simulink model "P702_NI_SoftECU"  (R2019a)
settings: Solver=ode1  StartTime=0.0  StopTime=Inf  FixedStep=0.001  RelTol=1e-3  EnableMultiTasking=on
PreLoadFcn:
  | run '.\VeriStand_BlockSet\NIVeriStandAddPaths.m'
undefined symbols (not defined in the file or in its folder): magnitude
libraries: simulink x83, simulink_extras x1
(part 47 of 76)

== system P702_NI_SoftECU/Input/GWM-SCCM//PDB//RCM//GSM/Other_GWMTx/Driver_Dr_Stat_FD1 ==
  BLISLEDStatDriverSide : S-Function  Priority=1  FunctionName=NIVeriStandIO  Parameters=width dtype portnum stime stype btype  SFunctionDeploymentMode=off  EnableBusSupport=off  mask(NI VeriStand Inport){portnum=1, width=-1, stime=-1, dtype=auto, stype=auto, btype=1}
      mask prompts: portnum "Port number:"; width "Port dimensions (-1 for dynamically sized):"; stime "Sample time (-1 for inherited):"; dtype "Data type:"; stype "Signal type:"; btype "Block type:"
      mask help: Use this inport on any level of nested subsystems to allow NI VeriStand software to map signals to it.
      mask init:
      | NIVeriStandIO_init;
      settings: CopyFcn=NIVeriStand_MDL_functions('', 'IO_copy');  DeleteFcn=NIVeriStand_MDL_functions('', 'IO_delete');  MoveFcn=set_param(gcb, 'Mask', 'on');
      mask Callback portnum: NIVeriStand_MDL_functions('', 'IO_setportnum');
      mask TypeOptions dtype: auto | double | single | int8 | uint8 | int16 | uint16 | int32 | uint32 | boolean
      mask Callback dtype: NIVeriStand_MDL_functions('', 'IO_booleansignal');
      mask TypeOptions stype: auto | real | complex
      mask Display:
      | patch([-x x], [-y y], [.90980 .81960 .32156]);
      | plot([xrad -x x xrad], [yrad -y y yrad]);
      | fprintf('NI In%d', portnum);
  Bus_Sig : BusCreator  Inputs=10
  ChildLckFdbckRd_B_Stat : S-Function  Priority=2  FunctionName=NIVeriStandIO  Parameters=width dtype portnum stime stype btype  SFunctionDeploymentMode=off  EnableBusSupport=off  mask(NI VeriStand Inport){portnum=2, width=-1, stime=-1, dtype=auto, stype=auto, btype=1}
      mask prompts: portnum "Port number:"; width "Port dimensions (-1 for dynamically sized):"; stime "Sample time (-1 for inherited):"; dtype "Data type:"; stype "Signal type:"; btype "Block type:"
      mask help: Use this inport on any level of nested subsystems to allow NI VeriStand software to map signals to it.
      mask init:
      | NIVeriStandIO_init;
      settings: CopyFcn=NIVeriStand_MDL_functions('', 'IO_copy');  DeleteFcn=NIVeriStand_MDL_functions('', 'IO_delete');  MoveFcn=set_param(gcb, 'Mask', 'on');
      mask Callback portnum: NIVeriStand_MDL_functions('', 'IO_setportnum');
      mask TypeOptions dtype: auto | double | single | int8 | uint8 | int16 | uint16 | int32 | uint32 | boolean
      mask Callback dtype: NIVeriStand_MDL_functions('', 'IO_booleansignal');
      mask TypeOptions stype: auto | real | complex
      mask Display:
      | patch([-x x], [-y y], [.90980 .81960 .32156]);
      | plot([xrad -x x xrad], [yrad -y y yrad]);
      | fprintf('NI In%d', portnum);
  ChildLckPw_D_Rq : S-Function  Priority=3  FunctionName=NIVeriStandIO  Parameters=width dtype portnum stime stype btype  SFunctionDeploymentMode=off  EnableBusSupport=off  mask(NI VeriStand Inport){portnum=3, width=-1, stime=-1, dtype=auto, stype=auto, btype=1}
      mask prompts: portnum "Port number:"; width "Port dimensions (-1 for dynamically sized):"; stime "Sample time (-1 for inherited):"; dtype "Data type:"; stype "Signal type:"; btype "Block type:"
      mask help: Use this inport on any level of nested subsystems to allow NI VeriStand software to map signals to it.
      mask init:
      | NIVeriStandIO_init;
      settings: CopyFcn=NIVeriStand_MDL_functions('', 'IO_copy');  DeleteFcn=NIVeriStand_MDL_functions('', 'IO_delete');  MoveFcn=set_param(gcb, 'Mask', 'on');
      mask Callback portnum: NIVeriStand_MDL_functions('', 'IO_setportnum');
      mask TypeOptions dtype: auto | double | single | int8 | uint8 | int16 | uint16 | int32 | uint32 | boolean
      mask Callback dtype: NIVeriStand_MDL_functions('', 'IO_booleansignal');
      mask TypeOptions stype: auto | real | complex
      mask Display:
      | patch([-x x], [-y y], [.90980 .81960 .32156]);
      | plot([xrad -x x xrad], [yrad -y y yrad]);
      | fprintf('NI In%d', portnum);
  ChildLckPw_N_Cnt : S-Function  Priority=4  FunctionName=NIVeriStandIO  Parameters=width dtype portnum stime stype btype  SFunctionDeploymentMode=off  EnableBusSupport=off  mask(NI VeriStand Inport){portnum=4, width=-1, stime=-1, dtype=auto, stype=auto, btype=1}
      mask prompts: portnum "Port number:"; width "Port dimensions (-1 for dynamically sized):"; stime "Sample time (-1 for inherited):"; dtype "Data type:"; stype "Signal type:"; btype "Block type:"
      mask help: Use this inport on any level of nested subsystems to allow NI VeriStand software to map signals to it.
      mask init:
      | NIVeriStandIO_init;
      settings: CopyFcn=NIVeriStand_MDL_functions('', 'IO_copy');  DeleteFcn=NIVeriStand_MDL_functions('', 'IO_delete');  MoveFcn=set_param(gcb, 'Mask', 'on');
      mask Callback portnum: NIVeriStand_MDL_functions('', 'IO_setportnum');
      mask TypeOptions dtype: auto | double | single | int8 | uint8 | int16 | uint16 | int32 | uint32 | boolean
      mask Callback dtype: NIVeriStand_MDL_functions('', 'IO_booleansignal');
      mask TypeOptions stype: auto | real | complex
      mask Display:
      | patch([-x x], [-y y], [.90980 .81960 .32156]);
      | plot([xrad -x x xrad], [yrad -y y yrad]);
      | fprintf('NI In%d', portnum);
  Driver_Lock_Sw_Cnt : S-Function  Priority=5  FunctionName=NIVeriStandIO  Parameters=width dtype portnum stime stype btype  SFunctionDeploymentMode=off  EnableBusSupport=off  mask(NI VeriStand Inport){portnum=5, width=-1, stime=-1, dtype=auto, stype=auto, btype=1}
      mask prompts: portnum "Port number:"; width "Port dimensions (-1 for dynamically sized):"; stime "Sample time (-1 for inherited):"; dtype "Data type:"; stype "Signal type:"; btype "Block type:"
      mask help: Use this inport on any level of nested subsystems to allow NI VeriStand software to map signals to it.
      mask init:
      | NIVeriStandIO_init;
      settings: CopyFcn=NIVeriStand_MDL_functions('', 'IO_copy');  DeleteFcn=NIVeriStand_MDL_functions('', 'IO_delete');  MoveFcn=set_param(gcb, 'Mask', 'on');
      mask Callback portnum: NIVeriStand_MDL_functions('', 'IO_setportnum');
      mask TypeOptions dtype: auto | double | single | int8 | uint8 | int16 | uint16 | int32 | uint32 | boolean
      mask Callback dtype: NIVeriStand_MDL_functions('', 'IO_booleansignal');
      mask TypeOptions stype: auto | real | complex
      mask Display:
      | patch([-x x], [-y y], [.90980 .81960 .32156]);
      | plot([xrad -x x xrad], [yrad -y y yrad]);
      | fprintf('NI In%d', portnum);
  Driver_Lock_Sw_Stat : S-Function  Priority=6  FunctionName=NIVeriStandIO  Parameters=width dtype portnum stime stype btype  SFunctionDeploymentMode=off  EnableBusSupport=off  mask(NI VeriStand Inport){portnum=6, width=-1, stime=-1, dtype=auto, stype=auto, btype=1}
      mask prompts: portnum "Port number:"; width "Port dimensions (-1 for dynamically sized):"; stime "Sample time (-1 for inherited):"; dtype "Data type:"; stype "Signal type:"; btype "Block type:"
      mask help: Use this inport on any level of nested subsystems to allow NI VeriStand software to map signals to it.
      mask init:
      | NIVeriStandIO_init;
      settings: CopyFcn=NIVeriStand_MDL_functions('', 'IO_copy');  DeleteFcn=NIVeriStand_MDL_functions('', 'IO_delete');  MoveFcn=set_param(gcb, 'Mask', 'on');
      mask Callback portnum: NIVeriStand_MDL_functions('', 'IO_setportnum');
      mask TypeOptions dtype: auto | double | single | int8 | uint8 | int16 | uint16 | int32 | uint32 | boolean
      mask Callback dtype: NIVeriStand_MDL_functions('', 'IO_booleansignal');
      mask TypeOptions stype: auto | real | complex
      mask Display:
      | patch([-x x], [-y y], [.90980 .81960 .32156]);
      | plot([xrad -x x xrad], [yrad -y y yrad]);
      | fprintf('NI In%d', portnum);
  KeyCylSwDrvDr_D_Stat : S-Function  Priority=7  FunctionName=NIVeriStandIO  Parameters=width dtype portnum stime stype btype  SFunctionDeploymentMode=off  EnableBusSupport=off  mask(NI VeriStand Inport){portnum=7, width=-1, stime=-1, dtype=auto, stype=auto, btype=1}
      mask prompts: portnum "Port number:"; width "Port dimensions (-1 for dynamically sized):"; stime "Sample time (-1 for inherited):"; dtype "Data type:"; stype "Signal type:"; btype "Block type:"
      mask help: Use this inport on any level of nested subsystems to allow NI VeriStand software to map signals to it.
      mask init:
      | NIVeriStandIO_init;
      settings: CopyFcn=NIVeriStand_MDL_functions('', 'IO_copy');  DeleteFcn=NIVeriStand_MDL_functions('', 'IO_delete');  MoveFcn=set_param(gcb, 'Mask', 'on');
      mask Callback portnum: NIVeriStand_MDL_functions('', 'IO_setportnum');
      mask TypeOptions dtype: auto | double | single | int8 | uint8 | int16 | uint16 | int32 | uint32 | boolean
      mask Callback dtype: NIVeriStand_MDL_functions('', 'IO_booleansignal');
      mask TypeOptions stype: auto | real | complex
      mask Display:
      | patch([-x x], [-y y], [.90980 .81960 .32156]);
      | plot([xrad -x x xrad], [yrad -y y yrad]);
      | fprintf('NI In%d', portnum);
  RollCodeDrvDrKeyCyl : S-Function  Priority=8  FunctionName=NIVeriStandIO  Parameters=width dtype portnum stime stype btype  SFunctionDeploymentMode=off  EnableBusSupport=off  mask(NI VeriStand Inport){portnum=8, width=-1, stime=-1, dtype=auto, stype=auto, btype=1}
      mask prompts: portnum "Port number:"; width "Port dimensions (-1 for dynamically sized):"; stime "Sample time (-1 for inherited):"; dtype "Data type:"; stype "Signal type:"; btype "Block type:"
      mask help: Use this inport on any level of nested subsystems to allow NI VeriStand software to map signals to it.
      mask init:
      | NIVeriStandIO_init;
      settings: CopyFcn=NIVeriStand_MDL_functions('', 'IO_copy');  DeleteFcn=NIVeriStand_MDL_functions('', 'IO_delete');  MoveFcn=set_param(gcb, 'Mask', 'on');
      mask Callback portnum: NIVeriStand_MDL_functions('', 'IO_setportnum');
      mask TypeOptions dtype: auto | double | single | int8 | uint8 | int16 | uint16 | int32 | uint32 | boolean
      mask Callback dtype: NIVeriStand_MDL_functions('', 'IO_booleansignal');
      mask TypeOptions stype: auto | real | complex
      mask Display:
      | patch([-x x], [-y y], [.90980 .81960 .32156]);
      | plot([xrad -x x xrad], [yrad -y y yrad]);
      | fprintf('NI In%d', portnum);
  RvrseMirrorChime_B_Rq : S-Function  Priority=9  FunctionName=NIVeriStandIO  Parameters=width dtype portnum stime stype btype  SFunctionDeploymentMode=off  EnableBusSupport=off  mask(NI VeriStand Inport){portnum=9, width=-1, stime=-1, dtype=auto, stype=auto, btype=1}
      mask prompts: portnum "Port number:"; width "Port dimensions (-1 for dynamically sized):"; stime "Sample time (-1 for inherited):"; dtype "Data type:"; stype "Signal type:"; btype "Block type:"
      mask help: Use this inport on any level of nested subsystems to allow NI VeriStand software to map signals to it.
      mask init:
      | NIVeriStandIO_init;
      settings: CopyFcn=NIVeriStand_MDL_functions('', 'IO_copy');  DeleteFcn=NIVeriStand_MDL_functions('', 'IO_delete');  MoveFcn=set_param(gcb, 'Mask', 'on');
      mask Callback portnum: NIVeriStand_MDL_functions('', 'IO_setportnum');
      mask TypeOptions dtype: auto | double | single | int8 | uint8 | int16 | uint16 | int32 | uint32 | boolean
      mask Callback dtype: NIVeriStand_MDL_functions('', 'IO_booleansignal');
      mask TypeOptions stype: auto | real | complex
      mask Display:
      | patch([-x x], [-y y], [.90980 .81960 .32156]);
      | plot([xrad -x x xrad], [yrad -y y yrad]);
      | fprintf('NI In%d', portnum);
  WndwDrvSide_D_Stat : S-Function  Priority=10  FunctionName=NIVeriStandIO  Parameters=width dtype portnum stime stype btype  SFunctionDeploymentMode=off  EnableBusSupport=off  mask(NI VeriStand Inport){portnum=10, width=-1, stime=-1, dtype=auto, stype=auto, btype=1}
      mask prompts: portnum "Port number:"; width "Port dimensions (-1 for dynamically sized):"; stime "Sample time (-1 for inherited):"; dtype "Data type:"; stype "Signal type:"; btype "Block type:"
      mask help: Use this inport on any level of nested subsystems to allow NI VeriStand software to map signals to it.
      mask init:
      | NIVeriStandIO_init;
      settings: CopyFcn=NIVeriStand_MDL_functions('', 'IO_copy');  DeleteFcn=NIVeriStand_MDL_functions('', 'IO_delete');  MoveFcn=set_param(gcb, 'Mask', 'on');
      mask Callback portnum: NIVeriStand_MDL_functions('', 'IO_setportnum');
      mask TypeOptions dtype: auto | double | single | int8 | uint8 | int16 | uint16 | int32 | uint32 | boolean
      mask Callback dtype: NIVeriStand_MDL_functions('', 'IO_booleansignal');
      mask TypeOptions stype: auto | real | complex
      mask Display:
      | patch([-x x], [-y y], [.90980 .81960 .32156]);
      | plot([xrad -x x xrad], [yrad -y y yrad]);
      | fprintf('NI In%d', portnum);
  Driver_Dr_Stat_FD1_332 : Outport
  wires:
  Bus_Sig/1 -> Driver_Dr_Stat_FD1_332/1  "Driver_Dr_Stat_FD1"
  BLISLEDStatDriverSide/1 -> Bus_Sig/1  "BLISLEDStatDriverSide"
  ChildLckFdbckRd_B_Stat/1 -> Bus_Sig/2  "ChildLckFdbckRd_B_Stat"
  ChildLckPw_D_Rq/1 -> Bus_Sig/3  "ChildLckPw_D_Rq"
  ChildLckPw_N_Cnt/1 -> Bus_Sig/4  "ChildLckPw_N_Cnt"
  Driver_Lock_Sw_Cnt/1 -> Bus_Sig/5  "Driver_Lock_Sw_Cnt"
  Driver_Lock_Sw_Stat/1 -> Bus_Sig/6  "Driver_Lock_Sw_Stat"
  KeyCylSwDrvDr_D_Stat/1 -> Bus_Sig/7  "KeyCylSwDrvDr_D_Stat"
  RollCodeDrvDrKeyCyl/1 -> Bus_Sig/8  "RollCodeDrvDrKeyCyl"
  RvrseMirrorChime_B_Rq/1 -> Bus_Sig/9  "RvrseMirrorChime_B_Rq"
  WndwDrvSide_D_Stat/1 -> Bus_Sig/10  "WndwDrvSide_D_Stat"

== system P702_NI_SoftECU/Input/GWM-SCCM//PDB//RCM//GSM/Other_GWMTx/Dsp_Request_Signals11_FD1 ==
  ApaMdeStat_D_RqDrv : Constant  Value=0
  ApaSwtch_D_RqMnu : Constant  Value=0
  Bus_Sig : BusCreator  Inputs=9
  CamAutoTowbarZoom : Constant  Value=0
  CamraOvrlDyn_D_Rq : Constant  Value=0
  CamraOvrlStat_D_Rq : Constant  Value=0
  CamraViewSplit_B_Rq : Constant  Value=0
  CamraZoomMan_D_Rq : Constant  Value=0
  DistanceBarSetting : Constant  Value=0
  PrkAidSwtch_D_RqMnu : Constant  Value=0
  Dsp_Request_Signals11_FD1_192 : Outport
  wires:
  Bus_Sig/1 -> Dsp_Request_Signals11_FD1_192/1  "Dsp_Request_Signals11_FD1_192"
  ApaMdeStat_D_RqDrv/1 -> Bus_Sig/1  "ApaMdeStat_D_RqDrv"
  ApaSwtch_D_RqMnu/1 -> Bus_Sig/2  "ApaSwtch_D_RqMnu"
  CamAutoTowbarZoom/1 -> Bus_Sig/3  "CamAutoTowbarZoom"
  CamraOvrlDyn_D_Rq/1 -> Bus_Sig/4  "CamraOvrlDyn_D_Rq"
  CamraOvrlStat_D_Rq/1 -> Bus_Sig/5  "CamraOvrlStat_D_Rq"
  CamraViewSplit_B_Rq/1 -> Bus_Sig/6  "CamraViewSplit_B_Rq"
  CamraZoomMan_D_Rq/1 -> Bus_Sig/7  "CamraZoomMan_D_Rq"
  DistanceBarSetting/1 -> Bus_Sig/8  "DistanceBarSetting"
  PrkAidSwtch_D_RqMnu/1 -> Bus_Sig/9  "PrkAidSwtch_D_RqMnu"

== system P702_NI_SoftECU/Input/GWM-SCCM//PDB//RCM//GSM/Other_GWMTx/ElecHorizon_Data1_FD1 ==
  Bus_Sig : BusCreator  Inputs=1
  EhData1_No_Actl : Constant  Value=0
  ElecHorizon_Data1_FD1_22E : Outport
  wires:
  Bus_Sig/1 -> ElecHorizon_Data1_FD1_22E/1  "ElecHorizon_Data1_FD1_22E"
  EhData1_No_Actl/1 -> Bus_Sig/1  "EhData1_No_Actl"

== system P702_NI_SoftECU/Input/GWM-SCCM//PDB//RCM//GSM/Other_GWMTx/ElecHorizon_Data2_FD1 ==
  Bus_Sig : BusCreator  Inputs=1
  EhData2_No_Actl : Constant  Value=0
  ElecHorizon_Data2_FD1_22F : Outport
  wires:
  Bus_Sig/1 -> ElecHorizon_Data2_FD1_22F/1  "ElecHorizon_Data2_FD1_22F"
  EhData2_No_Actl/1 -> Bus_Sig/1  "EhData2_No_Actl"

== system P702_NI_SoftECU/Input/GWM-SCCM//PDB//RCM//GSM/Other_GWMTx/FourByFourSwitchData_FD1 ==
  AwdLck_D_RqDrv : S-Function  Priority=1  FunctionName=NIVeriStandIO  Parameters=width dtype portnum stime stype btype  SFunctionDeploymentMode=off  EnableBusSupport=off  mask(NI VeriStand Inport){portnum=1, width=-1, stime=-1, dtype=auto, stype=auto, btype=1}
      mask prompts: portnum "Port number:"; width "Port dimensions (-1 for dynamically sized):"; stime "Sample time (-1 for inherited):"; dtype "Data type:"; stype "Signal type:"; btype "Block type:"
      mask help: Use this inport on any level of nested subsystems to allow NI VeriStand software to map signals to it.
      mask init:
      | NIVeriStandIO_init;
      settings: CopyFcn=NIVeriStand_MDL_functions('', 'IO_copy');  DeleteFcn=NIVeriStand_MDL_functions('', 'IO_delete');  MoveFcn=set_param(gcb, 'Mask', 'on');
      mask Callback portnum: NIVeriStand_MDL_functions('', 'IO_setportnum');
      mask TypeOptions dtype: auto | double | single | int8 | uint8 | int16 | uint16 | int32 | uint32 | boolean
      mask Callback dtype: NIVeriStand_MDL_functions('', 'IO_booleansignal');
      mask TypeOptions stype: auto | real | complex
      mask Display:
      | patch([-x x], [-y y], [.90980 .81960 .32156]);
      | plot([xrad -x x xrad], [yrad -y y yrad]);
      | fprintf('NI In%d', portnum);
  AwdMde_D_RqDrv : S-Function  Priority=2  FunctionName=NIVeriStandIO  Parameters=width dtype portnum stime stype btype  SFunctionDeploymentMode=off  EnableBusSupport=off  mask(NI VeriStand Inport){portnum=2, width=-1, stime=-1, dtype=auto, stype=auto, btype=1}
      mask prompts: portnum "Port number:"; width "Port dimensions (-1 for dynamically sized):"; stime "Sample time (-1 for inherited):"; dtype "Data type:"; stype "Signal type:"; btype "Block type:"
      mask help: Use this inport on any level of nested subsystems to allow NI VeriStand software to map signals to it.
      mask init:
      | NIVeriStandIO_init;
      settings: CopyFcn=NIVeriStand_MDL_functions('', 'IO_copy');  DeleteFcn=NIVeriStand_MDL_functions('', 'IO_delete');  MoveFcn=set_param(gcb, 'Mask', 'on');
      mask Callback portnum: NIVeriStand_MDL_functions('', 'IO_setportnum');
      mask TypeOptions dtype: auto | double | single | int8 | uint8 | int16 | uint16 | int32 | uint32 | boolean
      mask Callback dtype: NIVeriStand_MDL_functions('', 'IO_booleansignal');
      mask TypeOptions stype: auto | real | complex
      mask Display:
      | patch([-x x], [-y y], [.90980 .81960 .32156]);
      | plot([xrad -x x xrad], [yrad -y y yrad]);
      | fprintf('NI In%d', portnum);
  Bus_Sig : BusCreator  Inputs=7
  DrvSlipCtlMde_B_Rq3 : S-Function  Priority=3  FunctionName=NIVeriStandIO  Parameters=width dtype portnum stime stype btype  SFunctionDeploymentMode=off  EnableBusSupport=off  mask(NI VeriStand Inport){portnum=3, width=-1, stime=-1, dtype=auto, stype=auto, btype=1}
      mask prompts: portnum "Port number:"; width "Port dimensions (-1 for dynamically sized):"; stime "Sample time (-1 for inherited):"; dtype "Data type:"; stype "Signal type:"; btype "Block type:"
      mask help: Use this inport on any level of nested subsystems to allow NI VeriStand software to map signals to it.
      mask init:
      | NIVeriStandIO_init;
      settings: CopyFcn=NIVeriStand_MDL_functions('', 'IO_copy');  DeleteFcn=NIVeriStand_MDL_functions('', 'IO_delete');  MoveFcn=set_param(gcb, 'Mask', 'on');
      mask Callback portnum: NIVeriStand_MDL_functions('', 'IO_setportnum');
      mask TypeOptions dtype: auto | double | single | int8 | uint8 | int16 | uint16 | int32 | uint32 | boolean
      mask Callback dtype: NIVeriStand_MDL_functions('', 'IO_booleansignal');
      mask TypeOptions stype: auto | real | complex
      mask Display:
      | patch([-x x], [-y y], [.90980 .81960 .32156]);
      | plot([xrad -x x xrad], [yrad -y y yrad]);
      | fprintf('NI In%d', portnum);
  HdcSwtchPos_B_Actl : S-Function  Priority=4  FunctionName=NIVeriStandIO  Parameters=width dtype portnum stime stype btype  SFunctionDeploymentMode=off  EnableBusSupport=off  mask(NI VeriStand Inport){portnum=4, width=-1, stime=-1, dtype=auto, stype=auto, btype=1}
      mask prompts: portnum "Port number:"; width "Port dimensions (-1 for dynamically sized):"; stime "Sample time (-1 for inherited):"; dtype "Data type:"; stype "Signal type:"; btype "Block type:"
      mask help: Use this inport on any level of nested subsystems to allow NI VeriStand software to map signals to it.
      mask init:
      | NIVeriStandIO_init;
      settings: CopyFcn=NIVeriStand_MDL_functions('', 'IO_copy');  DeleteFcn=NIVeriStand_MDL_functions('', 'IO_delete');  MoveFcn=set_param(gcb, 'Mask', 'on');
      mask Callback portnum: NIVeriStand_MDL_functions('', 'IO_setportnum');
      mask TypeOptions dtype: auto | double | single | int8 | uint8 | int16 | uint16 | int32 | uint32 | boolean
      mask Callback dtype: NIVeriStand_MDL_functions('', 'IO_booleansignal');
      mask TypeOptions stype: auto | real | complex
      mask Display:
      | patch([-x x], [-y y], [.90980 .81960 .32156]);
      | plot([xrad -x x xrad], [yrad -y y yrad]);
      | fprintf('NI In%d', portnum);
  HybMdeSwtch_B_Rq : S-Function  Priority=5  FunctionName=NIVeriStandIO  Parameters=width dtype portnum stime stype btype  SFunctionDeploymentMode=off  EnableBusSupport=off  mask(NI VeriStand Inport){portnum=5, width=-1, stime=-1, dtype=auto, stype=auto, btype=1}
      mask prompts: portnum "Port number:"; width "Port dimensions (-1 for dynamically sized):"; stime "Sample time (-1 for inherited):"; dtype "Data type:"; stype "Signal type:"; btype "Block type:"
      mask help: Use this inport on any level of nested subsystems to allow NI VeriStand software to map signals to it.
      mask init:
      | NIVeriStandIO_init;
      settings: CopyFcn=NIVeriStand_MDL_functions('', 'IO_copy');  DeleteFcn=NIVeriStand_MDL_functions('', 'IO_delete');  MoveFcn=set_param(gcb, 'Mask', 'on');
      mask Callback portnum: NIVeriStand_MDL_functions('', 'IO_setportnum');
      mask TypeOptions dtype: auto | double | single | int8 | uint8 | int16 | uint16 | int32 | uint32 | boolean
      mask Callback dtype: NIVeriStand_MDL_functions('', 'IO_booleansignal');
      mask TypeOptions stype: auto | real | complex
      mask Display:
      | patch([-x x], [-y y], [.90980 .81960 .32156]);
      | plot([xrad -x x xrad], [yrad -y y yrad]);
      | fprintf('NI In%d', portnum);
  RearDiffLck_D_RqDrv : S-Function  Priority=6  FunctionName=NIVeriStandIO  Parameters=width dtype portnum stime stype btype  SFunctionDeploymentMode=off  EnableBusSupport=off  mask(NI VeriStand Inport){portnum=6, width=-1, stime=-1, dtype=auto, stype=auto, btype=1}
      mask prompts: portnum "Port number:"; width "Port dimensions (-1 for dynamically sized):"; stime "Sample time (-1 for inherited):"; dtype "Data type:"; stype "Signal type:"; btype "Block type:"
      mask help: Use this inport on any level of nested subsystems to allow NI VeriStand software to map signals to it.
      mask init:
      | NIVeriStandIO_init;
      settings: CopyFcn=NIVeriStand_MDL_functions('', 'IO_copy');  DeleteFcn=NIVeriStand_MDL_functions('', 'IO_delete');  MoveFcn=set_param(gcb, 'Mask', 'on');
      mask Callback portnum: NIVeriStand_MDL_functions('', 'IO_setportnum');
      mask TypeOptions dtype: auto | double | single | int8 | uint8 | int16 | uint16 | int32 | uint32 | boolean
      mask Callback dtype: NIVeriStand_MDL_functions('', 'IO_booleansignal');
      mask TypeOptions stype: auto | real | complex
      mask Display:
      | patch([-x x], [-y y], [.90980 .81960 .32156]);
      | plot([xrad -x x xrad], [yrad -y y yrad]);
      | fprintf('NI In%d', portnum);
  TrailCtlSwtch_B_Stat3 : S-Function  Priority=7  FunctionName=NIVeriStandIO  Parameters=width dtype portnum stime stype btype  SFunctionDeploymentMode=off  EnableBusSupport=off  mask(NI VeriStand Inport){portnum=7, width=-1, stime=-1, dtype=auto, stype=auto, btype=1}
      mask prompts: portnum "Port number:"; width "Port dimensions (-1 for dynamically sized):"; stime "Sample time (-1 for inherited):"; dtype "Data type:"; stype "Signal type:"; btype "Block type:"
      mask help: Use this inport on any level of nested subsystems to allow NI VeriStand software to map signals to it.
      mask init:
      | NIVeriStandIO_init;
      settings: CopyFcn=NIVeriStand_MDL_functions('', 'IO_copy');  DeleteFcn=NIVeriStand_MDL_functions('', 'IO_delete');  MoveFcn=set_param(gcb, 'Mask', 'on');
      mask Callback portnum: NIVeriStand_MDL_functions('', 'IO_setportnum');
      mask TypeOptions dtype: auto | double | single | int8 | uint8 | int16 | uint16 | int32 | uint32 | boolean
      mask Callback dtype: NIVeriStand_MDL_functions('', 'IO_booleansignal');
      mask TypeOptions stype: auto | real | complex
      mask Display:
      | patch([-x x], [-y y], [.90980 .81960 .32156]);
      | plot([xrad -x x xrad], [yrad -y y yrad]);
      | fprintf('NI In%d', portnum);
  FourByFourSwitchData_FD1_460 : Outport
  wires:
  Bus_Sig/1 -> FourByFourSwitchData_FD1_460/1  "FourByFourSwitchData_FD1_460"
  AwdLck_D_RqDrv/1 -> Bus_Sig/1  "AwdLck_D_RqDrv"
  AwdMde_D_RqDrv/1 -> Bus_Sig/2  "AwdMde_D_RqDrv"
  DrvSlipCtlMde_B_Rq3/1 -> Bus_Sig/3  "DrvSlipCtlMde_B_Rq3"
  HdcSwtchPos_B_Actl/1 -> Bus_Sig/4  "HdcSwtchPos_B_Actl"
  HybMdeSwtch_B_Rq/1 -> Bus_Sig/5  "HybMdeSwtch_B_Rq"
  RearDiffLck_D_RqDrv/1 -> Bus_Sig/6  "RearDiffLck_D_RqDrv"
  TrailCtlSwtch_B_Stat3/1 -> Bus_Sig/7  "TrailCtlSwtch_B_Stat3"

== system P702_NI_SoftECU/Input/GWM-SCCM//PDB//RCM//GSM/Other_GWMTx/Front_Distance_Req_FD1 ==
  Bus_Sig : BusCreator  Inputs=17
  FdsmTrgCntr_B_Actl : Constant  Value=0
  FdsmTrgDist_L_Actl : Constant  Value=0
  FdsmTrgLeft_B_Actl : Constant  Value=0
  FdsmTrgRight_B_Actl : Constant  Value=0
  LscmbbBaSens_D_Rq : Constant  Value=0
  LscmbbBlck_B_Actl : Constant  Value=0
  LscmbbBrkDecel_A_Rq : Constant  Value=0
  LscmbbBrkDecel_B_Enbl : Constant  Value=0
  LscmbbBrkDecel_No_Cnt : Constant  Value=0
  LscmbbBrkDecel_No_Cs : Constant  Value=0
  LscmbbBrkPrchg_D_Rq : Constant  Value=0
  LscmbbDeny_B_Actl : Constant  Value=0
  LscmbbEngTqMn_B_Rq : Constant  Value=0
  LscmbbMsgTxt_D_Rq : Constant  Value=0
  LscmbbPostEvnt_B_Dsply : Constant  Value=0
  LscmbbSrvcRqd_B_Rq : Constant  Value=0
  WndwFrontHeat_B_Rq : Constant  Value=0
  Front_Distance_Req_FD1_339 : Outport
  wires:
  Bus_Sig/1 -> Front_Distance_Req_FD1_339/1  "Front_Distance_Req_FD1_339"
  FdsmTrgCntr_B_Actl/1 -> Bus_Sig/1  "FdsmTrgCntr_B_Actl"
  FdsmTrgDist_L_Actl/1 -> Bus_Sig/2  "FdsmTrgDist_L_Actl"
  FdsmTrgLeft_B_Actl/1 -> Bus_Sig/3  "FdsmTrgLeft_B_Actl"
  FdsmTrgRight_B_Actl/1 -> Bus_Sig/4  "FdsmTrgRight_B_Actl"
  LscmbbBaSens_D_Rq/1 -> Bus_Sig/5  "LscmbbBaSens_D_Rq"
  LscmbbBlck_B_Actl/1 -> Bus_Sig/6  "LscmbbBlck_B_Actl"
  LscmbbBrkDecel_A_Rq/1 -> Bus_Sig/7  "LscmbbBrkDecel_A_Rq"
  LscmbbBrkDecel_B_Enbl/1 -> Bus_Sig/8  "LscmbbBrkDecel_B_Enbl"
  LscmbbBrkDecel_No_Cnt/1 -> Bus_Sig/9  "LscmbbBrkDecel_No_Cnt"
  LscmbbBrkDecel_No_Cs/1 -> Bus_Sig/10  "LscmbbBrkDecel_No_Cs"
  LscmbbBrkPrchg_D_Rq/1 -> Bus_Sig/11  "LscmbbBrkPrchg_D_Rq"
  LscmbbDeny_B_Actl/1 -> Bus_Sig/12  "LscmbbDeny_B_Actl"
  LscmbbEngTqMn_B_Rq/1 -> Bus_Sig/13  "LscmbbEngTqMn_B_Rq"
  LscmbbMsgTxt_D_Rq/1 -> Bus_Sig/14  "LscmbbMsgTxt_D_Rq"
  LscmbbPostEvnt_B_Dsply/1 -> Bus_Sig/15  "LscmbbPostEvnt_B_Dsply"
  LscmbbSrvcRqd_B_Rq/1 -> Bus_Sig/16  "LscmbbSrvcRqd_B_Rq"
  WndwFrontHeat_B_Rq/1 -> Bus_Sig/17  "WndwFrontHeat_B_Rq"

== system P702_NI_SoftECU/Input/GWM-SCCM//PDB//RCM//GSM/Other_GWMTx/GGCC_Config_Mgmt_ID_1_FD1 ==
  Bus_Sig : BusCreator  Inputs=1
  VehicleGGCCData : Constant  Value=0
  GGCC_Config_Mgmt_ID_1_FD1_40A : Outport
  wires:
  Bus_Sig/1 -> GGCC_Config_Mgmt_ID_1_FD1_40A/1  "GGCC_Config_Mgmt_ID_1_FD1_40A"
  VehicleGGCCData/1 -> Bus_Sig/1  "VehicleGGCCData"

== system P702_NI_SoftECU/Input/GWM-SCCM//PDB//RCM//GSM/Other_GWMTx/GWM_AutoSar_NetMgmt_FD1 ==
  Bus_Sig : BusCreator  Inputs=8
  GWM_AutoSarNMControl : Constant  Value=0
  GWM_AutoSarNMNodeId : Constant  Value=158
  GWM_AutoSarNMReserved{1..4} (4 alike) : Constant  Value=255
  GWM_GWNMProxy : Constant  Value=255
  GWM_GWOnBoardTester : Constant  Value=255
  GWM_AutoSar_NetMgmt_FD1_59E : Outport
  wires:
  Bus_Sig/1 -> GWM_AutoSar_NetMgmt_FD1_59E/1  "GWM_AutoSar_NetMgmt_FD1_59E"
  GWM_AutoSarNMControl/1 -> Bus_Sig/1  "GWM_AutoSarNMControl"
  GWM_AutoSarNMNodeId/1 -> Bus_Sig/2  "GWM_AutoSarNMNodeId"
  GWM_AutoSarNMReserved1/1 -> Bus_Sig/3  "GWM_AutoSarNMReserved1"
  GWM_AutoSarNMReserved2/1 -> Bus_Sig/4  "GWM_AutoSarNMReserved2"
  GWM_AutoSarNMReserved3/1 -> Bus_Sig/5  "GWM_AutoSarNMReserved3"
  GWM_AutoSarNMReserved4/1 -> Bus_Sig/6  "GWM_AutoSarNMReserved4"
  GWM_GWNMProxy/1 -> Bus_Sig/7  "GWM_GWNMProxy"
  GWM_GWOnBoardTester/1 -> Bus_Sig/8  "GWM_GWOnBoardTester"

== system P702_NI_SoftECU/Input/GWM-SCCM//PDB//RCM//GSM/Other_GWMTx/GlobalClock_Data_FD1 ==
  Bus_Sig : BusCreator  Inputs=5
  GlblClkDay_No_Actl : Constant  Value=0
  GlblClkHr_No_Actl : Constant  Value=0
  GlblClkMnte_No_Actl : Constant  Value=0
  GlblClkScnd_No_Actl : Constant  Value=0
  GlblClkYr_No_Actl : Constant  Value=0
  GlobalClock_Data_FD1_84 : Outport
  wires:
  Bus_Sig/1 -> GlobalClock_Data_FD1_84/1  "GlobalClock_Data_FD1_84"
  GlblClkDay_No_Actl/1 -> Bus_Sig/1  "GlblClkDay_No_Actl"
  GlblClkHr_No_Actl/1 -> Bus_Sig/2  "GlblClkHr_No_Actl"
  GlblClkMnte_No_Actl/1 -> Bus_Sig/3  "GlblClkMnte_No_Actl"
  GlblClkScnd_No_Actl/1 -> Bus_Sig/4  "GlblClkScnd_No_Actl"
  GlblClkYr_No_Actl/1 -> Bus_Sig/5  "GlblClkYr_No_Actl"

== system P702_NI_SoftECU/Input/GWM-SCCM//PDB//RCM//GSM/Other_GWMTx/Global_PATS_Cntrl_Info_FD1 ==
  Bus_Sig : BusCreator  Inputs=2
  immoControlCmd_T1 : Constant  Value=0
  immoControlData_T1 : Constant  Value=0
  Global_PATS_Cntrl_Info_FD1_41 : Outport
  wires:
  Bus_Sig/1 -> Global_PATS_Cntrl_Info_FD1_41/1  "Global_PATS_Cntrl_Info_FD1_41"
  immoControlCmd_T1/1 -> Bus_Sig/1  "immoControlCmd_T1"
  immoControlData_T1/1 -> Bus_Sig/2  "immoControlData_T1"

== system P702_NI_SoftECU/Input/GWM-SCCM//PDB//RCM//GSM/Other_GWMTx/IPC_Infotainment_FD1 ==
  BeltminderAudioMute : S-Function  Priority=1  FunctionName=NIVeriStandIO  Parameters=width dtype portnum stime stype btype  SFunctionDeploymentMode=off  EnableBusSupport=off  mask(NI VeriStand Inport){portnum=1, width=-1, stime=-1, dtype=auto, stype=auto, btype=1}
      mask prompts: portnum "Port number:"; width "Port dimensions (-1 for dynamically sized):"; stime "Sample time (-1 for inherited):"; dtype "Data type:"; stype "Signal type:"; btype "Block type:"
      mask help: Use this inport on any level of nested subsystems to allow NI VeriStand software to map signals to it.
      mask init:
      | NIVeriStandIO_init;
      settings: CopyFcn=NIVeriStand_MDL_functions('', 'IO_copy');  DeleteFcn=NIVeriStand_MDL_functions('', 'IO_delete');  MoveFcn=set_param(gcb, 'Mask', 'on');
      mask Callback portnum: NIVeriStand_MDL_functions('', 'IO_setportnum');
      mask TypeOptions dtype: auto | double | single | int8 | uint8 | int16 | uint16 | int32 | uint32 | boolean
      mask Callback dtype: NIVeriStand_MDL_functions('', 'IO_booleansignal');
      mask TypeOptions stype: auto | real | complex
      mask Display:
      | patch([-x x], [-y y], [.90980 .81960 .32156]);
      | plot([xrad -x x xrad], [yrad -y y yrad]);
      | fprintf('NI In%d', portnum);
  Bus_Sig : BusCreator  Inputs=8
  Chime_Source : S-Function  Priority=2  FunctionName=NIVeriStandIO  Parameters=width dtype portnum stime stype btype  SFunctionDeploymentMode=off  EnableBusSupport=off  mask(NI VeriStand Inport){portnum=2, width=-1, stime=-1, dtype=auto, stype=auto, btype=1}
      mask prompts: portnum "Port number:"; width "Port dimensions (-1 for dynamically sized):"; stime "Sample time (-1 for inherited):"; dtype "Data type:"; stype "Signal type:"; btype "Block type:"
      mask help: Use this inport on any level of nested subsystems to allow NI VeriStand software to map signals to it.
      mask init:
      | NIVeriStandIO_init;
      settings: CopyFcn=NIVeriStand_MDL_functions('', 'IO_copy');  DeleteFcn=NIVeriStand_MDL_functions('', 'IO_delete');  MoveFcn=set_param(gcb, 'Mask', 'on');
      mask Callback portnum: NIVeriStand_MDL_functions('', 'IO_setportnum');
      mask TypeOptions dtype: auto | double | single | int8 | uint8 | int16 | uint16 | int32 | uint32 | boolean
      mask Callback dtype: NIVeriStand_MDL_functions('', 'IO_booleansignal');
      mask TypeOptions stype: auto | real | complex
      mask Display:
      | patch([-x x], [-y y], [.90980 .81960 .32156]);
      | plot([xrad -x x xrad], [yrad -y y yrad]);
      | fprintf('NI In%d', portnum);
  HdcOn_B_Rq : S-Function  Priority=3  FunctionName=NIVeriStandIO  Parameters=width dtype portnum stime stype btype  SFunctionDeploymentMode=off  EnableBusSupport=off  mask(NI VeriStand Inport){portnum=3, width=-1, stime=-1, dtype=auto, stype=auto, btype=1}
      mask prompts: portnum "Port number:"; width "Port dimensions (-1 for dynamically sized):"; stime "Sample time (-1 for inherited):"; dtype "Data type:"; stype "Signal type:"; btype "Block type:"
      mask help: Use this inport on any level of nested subsystems to allow NI VeriStand software to map signals to it.
      mask init:
      | NIVeriStandIO_init;
      settings: CopyFcn=NIVeriStand_MDL_functions('', 'IO_copy');  DeleteFcn=NIVeriStand_MDL_functions('', 'IO_delete');  MoveFcn=set_param(gcb, 'Mask', 'on');
      mask Callback portnum: NIVeriStand_MDL_functions('', 'IO_setportnum');
      mask TypeOptions dtype: auto | double | single | int8 | uint8 | int16 | uint16 | int32 | uint32 | boolean
      mask Callback dtype: NIVeriStand_MDL_functions('', 'IO_booleansignal');
      mask TypeOptions stype: auto | real | complex
      mask Display:
      | patch([-x x], [-y y], [.90980 .81960 .32156]);
      | plot([xrad -x x xrad], [yrad -y y yrad]);
      | fprintf('NI In%d', portnum);
  IPC_Attn_Info_Audio : S-Function  Priority=4  FunctionName=NIVeriStandIO  Parameters=width dtype portnum stime stype btype  SFunctionDeploymentMode=off  EnableBusSupport=off  mask(NI VeriStand Inport){portnum=4, width=-1, stime=-1, dtype=auto, stype=auto, btype=1}
      mask prompts: portnum "Port number:"; width "Port dimensions (-1 for dynamically sized):"; stime "Sample time (-1 for inherited):"; dtype "Data type:"; stype "Signal type:"; btype "Block type:"
      mask help: Use this inport on any level of nested subsystems to allow NI VeriStand software to map signals to it.
      mask init:
      | NIVeriStandIO_init;
      settings: CopyFcn=NIVeriStand_MDL_functions('', 'IO_copy');  DeleteFcn=NIVeriStand_MDL_functions('', 'IO_delete');  MoveFcn=set_param(gcb, 'Mask', 'on');
      mask Callback portnum: NIVeriStand_MDL_functions('', 'IO_setportnum');
      mask TypeOptions dtype: auto | double | single | int8 | uint8 | int16 | uint16 | int32 | uint32 | boolean
      mask Callback dtype: NIVeriStand_MDL_functions('', 'IO_booleansignal');
      mask TypeOptions stype: auto | real | complex
      mask Display:
      | patch([-x x], [-y y], [.90980 .81960 .32156]);
      | plot([xrad -x x xrad], [yrad -y y yrad]);
      | fprintf('NI In%d', portnum);
  IPC_MyKeyVolLimit_St : S-Function  Priority=5  FunctionName=NIVeriStandIO  Parameters=width dtype portnum stime stype btype  SFunctionDeploymentMode=off  EnableBusSupport=off  mask(NI VeriStand Inport){portnum=5, width=-1, stime=-1, dtype=auto, stype=auto, btype=1}
      mask prompts: portnum "Port number:"; width "Port dimensions (-1 for dynamically sized):"; stime "Sample time (-1 for inherited):"; dtype "Data type:"; stype "Signal type:"; btype "Block type:"
      mask help: Use this inport on any level of nested subsystems to allow NI VeriStand software to map signals to it.
      mask init:
      | NIVeriStandIO_init;
      settings: CopyFcn=NIVeriStand_MDL_functions('', 'IO_copy');  DeleteFcn=NIVeriStand_MDL_functions('', 'IO_delete');  MoveFcn=set_param(gcb, 'Mask', 'on');
      mask Callback portnum: NIVeriStand_MDL_functions('', 'IO_setportnum');
      mask TypeOptions dtype: auto | double | single | int8 | uint8 | int16 | uint16 | int32 | uint32 | boolean
      mask Callback dtype: NIVeriStand_MDL_functions('', 'IO_booleansignal');
      mask TypeOptions stype: auto | real | complex
      mask Display:
      | patch([-x x], [-y y], [.90980 .81960 .32156]);
      | plot([xrad -x x xrad], [yrad -y y yrad]);
      | fprintf('NI In%d', portnum);
  IPC_New_Attn_Event : S-Function  Priority=6  FunctionName=NIVeriStandIO  Parameters=width dtype portnum stime stype btype  SFunctionDeploymentMode=off  EnableBusSupport=off  mask(NI VeriStand Inport){portnum=6, width=-1, stime=-1, dtype=auto, stype=auto, btype=1}
      mask prompts: portnum "Port number:"; width "Port dimensions (-1 for dynamically sized):"; stime "Sample time (-1 for inherited):"; dtype "Data type:"; stype "Signal type:"; btype "Block type:"
      mask help: Use this inport on any level of nested subsystems to allow NI VeriStand software to map signals to it.
      mask init:
      | NIVeriStandIO_init;
      settings: CopyFcn=NIVeriStand_MDL_functions('', 'IO_copy');  DeleteFcn=NIVeriStand_MDL_functions('', 'IO_delete');  MoveFcn=set_param(gcb, 'Mask', 'on');
      mask Callback portnum: NIVeriStand_MDL_functions('', 'IO_setportnum');
      mask TypeOptions dtype: auto | double | single | int8 | uint8 | int16 | uint16 | int32 | uint32 | boolean
      mask Callback dtype: NIVeriStand_MDL_functions('', 'IO_booleansignal');
      mask TypeOptions stype: auto | real | complex
      mask Display:
      | patch([-x x], [-y y], [.90980 .81960 .32156]);
      | plot([xrad -x x xrad], [yrad -y y yrad]);
      | fprintf('NI In%d', portnum);
  Power_Up_Chime_Modules : S-Function  Priority=7  FunctionName=NIVeriStandIO  Parameters=width dtype portnum stime stype btype  SFunctionDeploymentMode=off  EnableBusSupport=off  mask(NI VeriStand Inport){portnum=7, width=-1, stime=-1, dtype=auto, stype=auto, btype=1}
      mask prompts: portnum "Port number:"; width "Port dimensions (-1 for dynamically sized):"; stime "Sample time (-1 for inherited):"; dtype "Data type:"; stype "Signal type:"; btype "Block type:"
      mask help: Use this inport on any level of nested subsystems to allow NI VeriStand software to map signals to it.
      mask init:
      | NIVeriStandIO_init;
      settings: CopyFcn=NIVeriStand_MDL_functions('', 'IO_copy');  DeleteFcn=NIVeriStand_MDL_functions('', 'IO_delete');  MoveFcn=set_param(gcb, 'Mask', 'on');
      mask Callback portnum: NIVeriStand_MDL_functions('', 'IO_setportnum');
      mask TypeOptions dtype: auto | double | single | int8 | uint8 | int16 | uint16 | int32 | uint32 | boolean
      mask Callback dtype: NIVeriStand_MDL_functions('', 'IO_booleansignal');
      mask TypeOptions stype: auto | real | complex
      mask Display:
      | patch([-x x], [-y y], [.90980 .81960 .32156]);
      | plot([xrad -x x xrad], [yrad -y y yrad]);
      | fprintf('NI In%d', portnum);
  Veh_V2_Dsply : S-Function  Priority=8  FunctionName=NIVeriStandIO  Parameters=width dtype portnum stime stype btype  SFunctionDeploymentMode=off  EnableBusSupport=off  mask(NI VeriStand Inport){portnum=8, width=-1, stime=-1, dtype=auto, stype=auto, btype=1}
      mask prompts: portnum "Port number:"; width "Port dimensions (-1 for dynamically sized):"; stime "Sample time (-1 for inherited):"; dtype "Data type:"; stype "Signal type:"; btype "Block type:"
      mask help: Use this inport on any level of nested subsystems to allow NI VeriStand software to map signals to it.
      mask init:
      | NIVeriStandIO_init;
      settings: CopyFcn=NIVeriStand_MDL_functions('', 'IO_copy');  DeleteFcn=NIVeriStand_MDL_functions('', 'IO_delete');  MoveFcn=set_param(gcb, 'Mask', 'on');
      mask Callback portnum: NIVeriStand_MDL_functions('', 'IO_setportnum');
      mask TypeOptions dtype: auto | double | single | int8 | uint8 | int16 | uint16 | int32 | uint32 | boolean
      mask Callback dtype: NIVeriStand_MDL_functions('', 'IO_booleansignal');
      mask TypeOptions stype: auto | real | complex
      mask Display:
      | patch([-x x], [-y y], [.90980 .81960 .32156]);
      | plot([xrad -x x xrad], [yrad -y y yrad]);
      | fprintf('NI In%d', portnum);
  IPC_Infotainment_FD1_225 : Outport
  wires:
  Bus_Sig/1 -> IPC_Infotainment_FD1_225/1  "IPC_Infotainment_FD1_225"
  BeltminderAudioMute/1 -> Bus_Sig/1  "BeltminderAudioMute"
  Chime_Source/1 -> Bus_Sig/2  "Chime_Source"
  HdcOn_B_Rq/1 -> Bus_Sig/3  "HdcOn_B_Rq"
  IPC_Attn_Info_Audio/1 -> Bus_Sig/4  "IPC_Attn_Info_Audio"
  IPC_MyKeyVolLimit_St/1 -> Bus_Sig/5  "IPC_MyKeyVolLimit_St"
  IPC_New_Attn_Event/1 -> Bus_Sig/6  "IPC_New_Attn_Event"
  Power_Up_Chime_Modules/1 -> Bus_Sig/7  "Power_Up_Chime_Modules"
  Veh_V2_Dsply/1 -> Bus_Sig/8  "Veh_V2_Dsply"

== system P702_NI_SoftECU/Input/GWM-SCCM//PDB//RCM//GSM/Other_GWMTx/IPC_Send_Signals_2_FD1 ==
  Bus_Sig : BusCreator  Inputs=3
  ElLongTerm_L_Dsply : Constant  Value=0
  ElTrip_L_Dsply : Constant  Value=0
  FuelRange_L_Dsply : Constant  Value=0
  IPC_Send_Signals_2_FD1_318 : Outport
  wires:
  Bus_Sig/1 -> IPC_Send_Signals_2_FD1_318/1  "IPC_Send_Signals_2_FD1_318"
  ElLongTerm_L_Dsply/1 -> Bus_Sig/1  "ElLongTerm_L_Dsply"
  ElTrip_L_Dsply/1 -> Bus_Sig/2  "ElTrip_L_Dsply"
  FuelRange_L_Dsply/1 -> Bus_Sig/3  "FuelRange_L_Dsply"

== system P702_NI_SoftECU/Input/GWM-SCCM//PDB//RCM//GSM/Other_GWMTx/MHT_EV_Wakeup_FD1 ==
  BattChlrSov_B_Rq : Constant  Value=0
  BattChrgTrgtSoC_D_Rq : Constant  Value=0
  BattTracDrvSustn_B_Rq : Constant  Value=0
  BrkAppl_D_RqPt : Constant  Value=0
  Bus_Sig : BusCreator  Inputs=11
  CabnEvapSovFront_B_Rq : Constant  Value=0
  CabnEvapSovRear_B_Rq : Constant  Value=0
  HeatCoreSovRear_B_Rq : Constant  Value=0
  HtrnClntFlw_D_Rq : Constant  Value=0
  HtrnCnnctPwr_B_Stat : Constant  Value=0
  HtrnDcdcDis_B_Rq : Constant  Value=0
  PtcHtr_D_Stat : Constant  Value=0
  MHT_EV_Wakeup_FD1_478 : Outport
  wires:
  Bus_Sig/1 -> MHT_EV_Wakeup_FD1_478/1  "MHT_EV_Wakeup_FD1_478"
  BattChlrSov_B_Rq/1 -> Bus_Sig/1  "BattChlrSov_B_Rq"
  BattChrgTrgtSoC_D_Rq/1 -> Bus_Sig/2  "BattChrgTrgtSoC_D_Rq"
  BattTracDrvSustn_B_Rq/1 -> Bus_Sig/3  "BattTracDrvSustn_B_Rq"
  BrkAppl_D_RqPt/1 -> Bus_Sig/4  "BrkAppl_D_RqPt"
  CabnEvapSovFront_B_Rq/1 -> Bus_Sig/5  "CabnEvapSovFront_B_Rq"
  CabnEvapSovRear_B_Rq/1 -> Bus_Sig/6  "CabnEvapSovRear_B_Rq"
  HeatCoreSovRear_B_Rq/1 -> Bus_Sig/7  "HeatCoreSovRear_B_Rq"
  HtrnClntFlw_D_Rq/1 -> Bus_Sig/8  "HtrnClntFlw_D_Rq"
  HtrnCnnctPwr_B_Stat/1 -> Bus_Sig/9  "HtrnCnnctPwr_B_Stat"
  HtrnDcdcDis_B_Rq/1 -> Bus_Sig/10  "HtrnDcdcDis_B_Rq"
  PtcHtr_D_Stat/1 -> Bus_Sig/11  "PtcHtr_D_Stat"
